simulink model "HVAC"  (R2021b)
settings: Solver=ode45  StartTime=0.0  StopTime=10  RelTol=1e-3
settings Model: Creator=raj  LastModifiedBy=akhileshraj

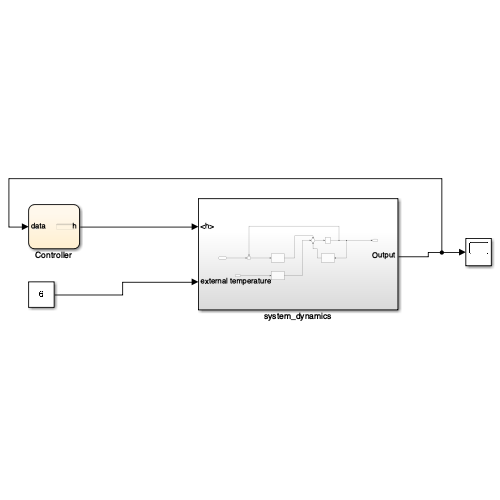
[thumbnail: Simulink's stored preview of the top-level diagram]
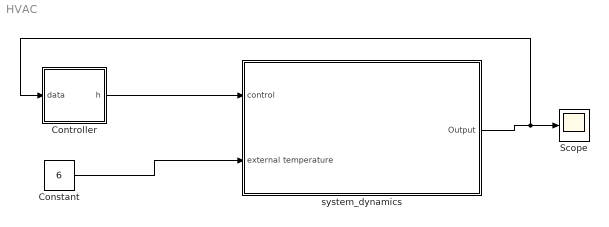
== system HVAC ==
  Constant : Constant  Value=6
  Controller : Stateflow chart  TreatAsAtomicUnit=on
  Scope : Scope
  system_dynamics : Subsystem
  wires:
  system_dynamics/1(Output) -> Controller/1(data), Scope/1
  Constant/1 -> system_dynamics/2(external temperature)
  Controller/1(h) -> system_dynamics/1(control)

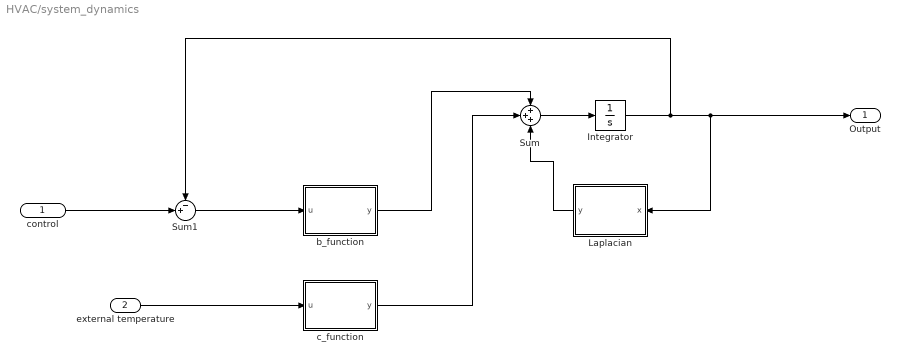
== system HVAC/system_dynamics ==
  control : Inport
  external temperature : Inport  Port=2
  Integrator : Integrator  InitialCondition=[16.5;16.5;16.5;16.5]
  Laplacian : MATLAB Function  TreatAsAtomicUnit=on
  Sum : Sum  Inputs=+++
  Sum1 : Sum  Inputs=-+|
  b_function : MATLAB Function  TreatAsAtomicUnit=on
  c_function : MATLAB Function  TreatAsAtomicUnit=on
  Output : Outport
  wires:
  c_function/1(y) -> Sum/2
  Sum/1 -> Integrator/1
  b_function/1(y) -> Sum/1
  Integrator/1 -> Sum1/1, Laplacian/1(x), Output/1
  Laplacian/1(y) -> Sum/3
  Sum1/1 -> b_function/1(u)
  control/1 -> Sum1/2
  external temperature/1 -> c_function/1(u)

== matlab function HVAC/system_dynamics/Laplacian ==
  data: x input; y output
function y = fcn(x)
A=[0,0.3,0.4,0.3;0.3,0,0.5,0;
    0.4,0.5,0,0.3;0.3,0,0.3,0];
degree = sum(A);
L = diag(degree)-A;
y = L*x;

== matlab function HVAC/system_dynamics/b_function ==
  data: u input; y output
function y = fcn(u)
b = [9,7,11,7]';
B = diag(b);
y = B*u;

== matlab function HVAC/system_dynamics/c_function ==
  data: u input; y output
function y = fcn(u)
c = [0.3,0.2,0.5,0.4]';
C = b;
y = C*u;

== stateflow chart HVAC/Controller ==
  state Room1
    state Heater1_Off
    state Heater1_On
    (default) -> Heater1_Off : {h(1)=0;}
    Heater1_Off -> Heater1_On : [x(1) <= on(1) && loc(1)==1]{h(1)=1;}
    Heater1_On -> Heater1_Off : [x(1) >= off(1) && loc(1)==0]{h(1)=0;}
  data: h output; data input
  function locator:
    | function locator()
    | for i = 1:4    
    |     if location(i) == 0 && x(i) <= get(i)
    |         for j = 1:4
    | 
    |             if i~=j && location(j) == 1 && x(j)-x(i) >= dif(i)
    |                 loc(i) = 1;
    |                 loc(j) = 0;
    |                 break
    |             end            
    |         end
    |     end
    | end
